simulink model "shooter"  (R2024a)
settings: Solver=VariableStepAuto  StartTime=0.0  StopTime=10.0  RelTol=1e-3
libraries: simulink x1
settings Model: Creator=micah  LastModifiedBy=micah

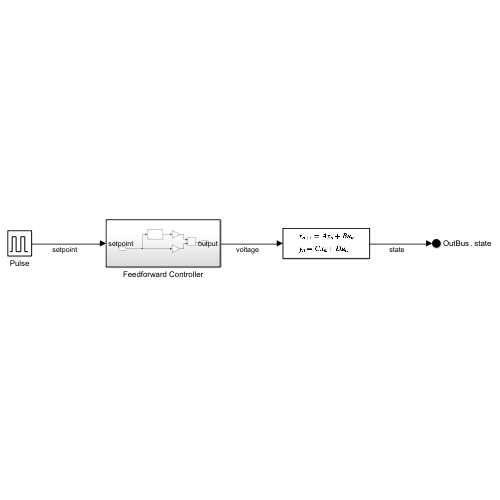
[thumbnail: Simulink's stored preview of the top-level diagram]
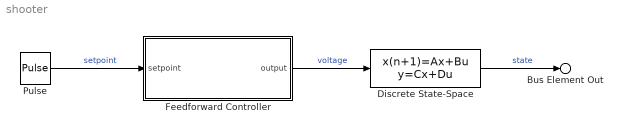
== system shooter ==
  Discrete State-Space : DiscreteStateSpace  SampleTime=-1
  Feedforward Controller : Subsystem
  Pulse : DiscretePulseGenerator  PulseType=Time based  Period=10  PulseWidth=5
  Bus Element Out : Outport  PortName=OutBus  Element=state
  wires:
  Pulse/1 -> Feedforward Controller/1(setpoint)  "setpoint"
  Feedforward Controller/1(output) -> Discrete State-Space/1  "voltage"
  Discrete State-Space/1 -> Bus Element Out/1  "state"

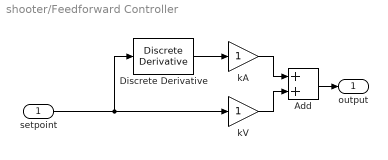
== system shooter/Feedforward Controller ==
  setpoint : Inport
  Add : Sum
  Discrete Derivative : simulink/Discrete/Discrete Derivative  gainval=1.0  ICPrevScaledInput=0.0  OutMin=[]  OutMax=[]  OutDataType=fixdt(1, 16)  OutScaling=2^-10  DoSatur=off
  kA : Gain
  kV : Gain
  output : Outport
  wires:
  kV/1 -> Add/2
  setpoint/1 -> kV/1, Discrete Derivative/1
  Discrete Derivative/1 -> kA/1
  kA/1 -> Add/1
  Add/1 -> output/1
